simulink model "TPS_SWC"  (R2022b)
settings: Solver=FixedStepDiscrete  StartTime=0.0  StopTime=10.0  FixedStep=0.1  RelTol=1e-3
libraries: pil_lib x1
settings Model: Creator=Abdelrhman Shaban  LastModifiedBy=Abdelrhman Shaban
settings OptimizationCC: DefaultParameterBehavior=Inlined  UseDivisionForNetSlopeComputation=on  GainParamInheritBuiltInType=on  UseFloatMulNetSlope=on  InlineInvariantSignals=on  PassReuseOutputArgsAs=Individual arguments  ZeroExternalMemoryAtStartup=off  ZeroInternalMemoryAtStartup=off  NoFixptDivByZeroProtection=on  EfficientFloat2IntCast=on  LifeSpan=1  OptimizeBlockOrder=speed  DifferentSizesBufferReuse=on  EfficientTunableParamExpr=on
settings DebuggingCC: ParameterTunabilityLossMsg=error
settings HardwareCC: ProdLongLongMode=on
settings SFSimCC: MATLABDynamicMemAlloc=off
settings RTWCC: Description=Embedded Coder  SystemTargetFile=ert.tlc  TemplateMakefile=ert_default_tmf  CreateSILPILBlock=SIL
settings CodeAppCC: ForceParamTrailComments=on  IgnoreCustomStorageClasses=off  OperatorAnnotations=on  SimulinkDataObjDesc=on  SFDataObjDesc=on  CustomSymbolStrGlobalVar=rt$N$M  CustomSymbolStrType=$N$M  CustomSymbolStrFcn=$N$M$F  CustomSymbolStrMacro=$N$M  InsertBlockDesc=on
settings ERTTargetCC: TargetLangStandard=C99 (ISO)  GenerateSampleERTMain=on  IncludeMdlTerminateFcn=off  CombineSignalStateStructs=on  SuppressErrorStatus=on  SupportAbsoluteTime=off  SupportComplex=off  InlinedParameterPlacement=NonHierarchical  ERTCustomFileTemplate=example_file_process.tlc  ERTFilePackagingFormat=CompactWithDataFile

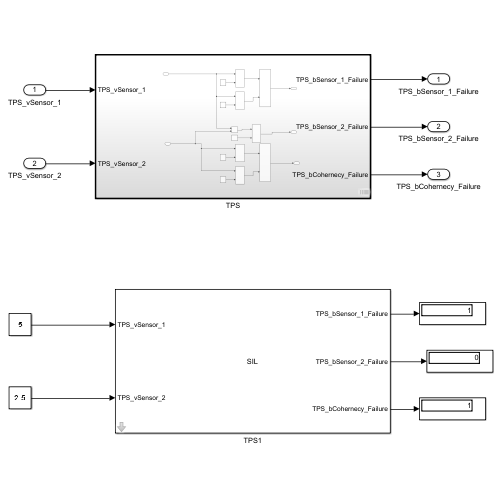
[thumbnail: Simulink's stored preview of the top-level diagram]
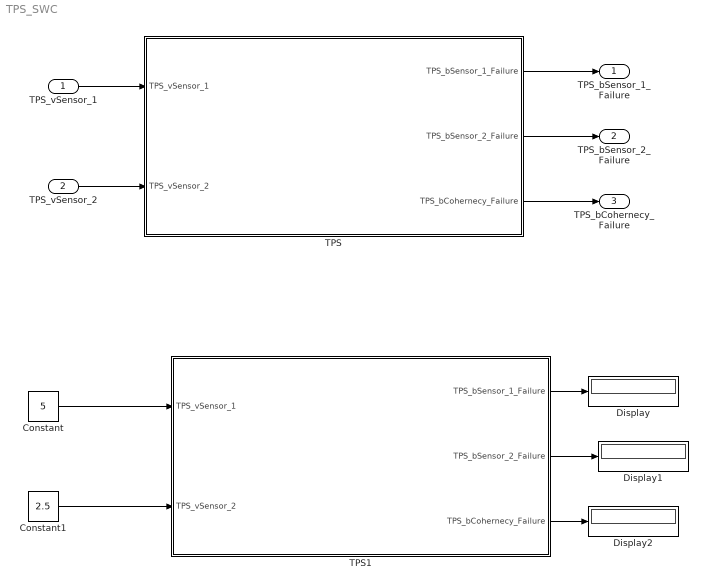
== system TPS_SWC ==
  TPS_vSensor_1 : Inport  OutDataTypeStr=single
  TPS_vSensor_2 : Inport  Port=2
  Constant : Constant  Value=5  OutDataTypeStr=single
  Constant1 : Constant  Value=2.5  OutDataTypeStr=single
  Display : Display
  Display1 : Display
  Display2 : Display
  TPS : Subsystem  TreatAsAtomicUnit=on
  TPS1 : Subsystem  Tag=__SL_testing_harness_stub_  DialogController=pil_create_dialog  LoadFcn=|
      | try
      |    if ~strcmp(rtw.pil.getPILVersion, '9.13 (R2022b)_15')
      |       set_param(gcb, 'DialogController', '');
      |       set_param(gcb, 'DialogControllerArgs', '');
      |    end
      | catch e
      |       set_param(gcb, 'DialogController', '');
      |       set_param(gcb, 'DialogControllerArgs', '');
      | end
      mask help: PIL:pil:XILBlockMaskDesc
      mask Display: disp('SIL');
  TPS_bSensor_1_Failure : Outport
  TPS_bSensor_2_Failure : Outport  Port=2
  TPS_bCohernecy_Failure : Outport  Port=3
  wires:
  TPS_vSensor_1/1 -> TPS/1(TPS_vSensor_1)
  TPS_vSensor_2/1 -> TPS/2(TPS_vSensor_2)
  TPS/1(TPS_bSensor_1_Failure) -> TPS_bSensor_1_Failure/1
  TPS/2(TPS_bSensor_2_Failure) -> TPS_bSensor_2_Failure/1
  TPS/3(TPS_bCohernecy_Failure) -> TPS_bCohernecy_Failure/1
  Constant/1 -> TPS1/1(TPS_vSensor_1)
  Constant1/1 -> TPS1/2(TPS_vSensor_2)
  TPS1/1(TPS_bSensor_1_Failure) -> Display/1
  TPS1/2(TPS_bSensor_2_Failure) -> Display1/1
  TPS1/3(TPS_bCohernecy_Failure) -> Display2/1

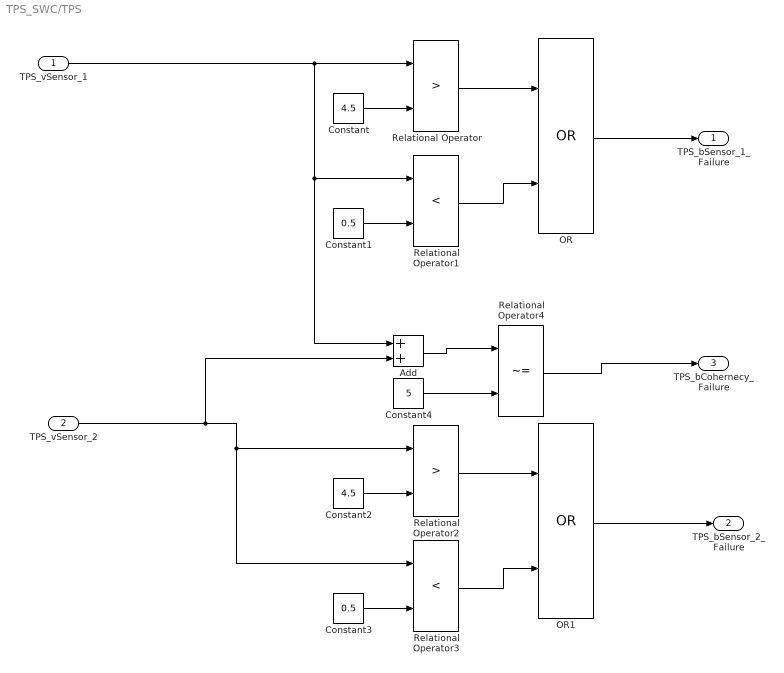
== system TPS_SWC/TPS ==
  TPS_vSensor_1 : Inport  OutDataTypeStr=single
  TPS_vSensor_2 : Inport  Port=2  OutDataTypeStr=single
  Add : Sum
  Constant : Constant  Value=4.5
  Constant1 : Constant  Value=0.5
  Constant2 : Constant  Value=4.5
  Constant3 : Constant  Value=0.5
  Constant4 : Constant  Value=5
  OR : Logic  Operator=OR  AllPortsSameDT=off  OutDataTypeStr=boolean
  OR1 : Logic  Operator=OR  AllPortsSameDT=off  OutDataTypeStr=boolean
  Relational Operator : RelationalOperator  Operator=>  OutDataTypeStr=boolean  RndMeth=Simplest  InputSameDT=off
  Relational Operator1 : RelationalOperator  Operator=<  OutDataTypeStr=boolean  RndMeth=Simplest  InputSameDT=off
  Relational Operator2 : RelationalOperator  Operator=>  OutDataTypeStr=boolean  RndMeth=Simplest  InputSameDT=off
  Relational Operator3 : RelationalOperator  Operator=<  OutDataTypeStr=boolean  RndMeth=Simplest  InputSameDT=off
  Relational Operator4 : RelationalOperator  Operator=~=  OutDataTypeStr=boolean  RndMeth=Simplest  InputSameDT=off
  TPS_bSensor_1_Failure : Outport  OutDataTypeStr=boolean
  TPS_bSensor_2_Failure : Outport  Port=2  OutDataTypeStr=boolean
  TPS_bCohernecy_Failure : Outport  Port=3  OutDataTypeStr=boolean
  wires:
  TPS_vSensor_1/1 -> Add/1, Relational Operator1/1, Relational Operator/1
  Constant/1 -> Relational Operator/2
  Constant1/1 -> Relational Operator1/2
  Relational Operator/1 -> OR/1
  Relational Operator1/1 -> OR/2
  OR/1 -> TPS_bSensor_1_Failure/1
  OR1/1 -> TPS_bSensor_2_Failure/1
  Relational Operator3/1 -> OR1/2
  Relational Operator2/1 -> OR1/1
  Constant3/1 -> Relational Operator3/2
  Constant2/1 -> Relational Operator2/2
  TPS_vSensor_2/1 -> Add/2, Relational Operator2/1, Relational Operator3/1
  Add/1 -> Relational Operator4/1
  Constant4/1 -> Relational Operator4/2
  Relational Operator4/1 -> TPS_bCohernecy_Failure/1

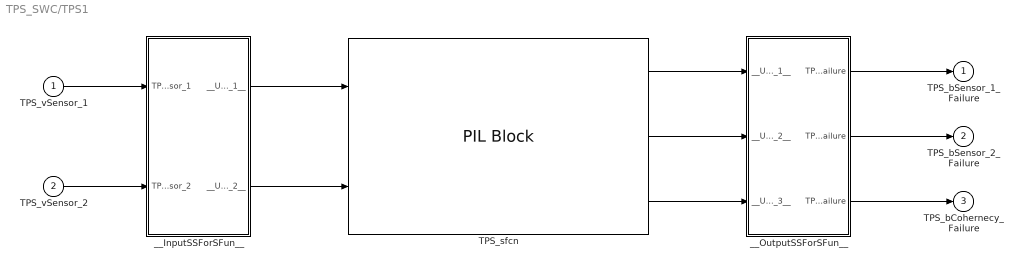
== system TPS_SWC/TPS1 ==
  TPS_vSensor_1 : Inport  OutDataTypeStr=single
  TPS_vSensor_2 : Inport  Port=2  OutDataTypeStr=single
  TPS_sfcn : pil_lib/PIL Block  SimulationMode=SIL  IsTopModelPIL=off  CodeDir=TPS_ert_rtw  AnchorDir=H:\AbdelrhmanWorkSpace\OSAcademy\Diploma\MBD_Diploma\6_System_Modeling\System_Modeling_Session_2\TechnicalPart\1_APP_Coherency  ConfigName=Software-in-the-Loop (SIL)  XrelIsTopModelCode=on  XrelIsReusable=off  XrelDWorkNames={}  XrelDWorkTypes={}  XrelModelArgVals={}  XrelOrderedParamNames={}
  __InputSSForSFun__ : Subsystem
  __OutputSSForSFun__ : Subsystem
  TPS_bSensor_1_Failure : Outport  OutDataTypeStr=boolean
  TPS_bSensor_2_Failure : Outport  Port=2  OutDataTypeStr=boolean
  TPS_bCohernecy_Failure : Outport  Port=3  OutDataTypeStr=boolean
  wires:
  __OutputSSForSFun__/3(TPS_bCohernecy_Failure) -> TPS_bCohernecy_Failure/1
  __OutputSSForSFun__/2(TPS_bSensor_2_Failure) -> TPS_bSensor_2_Failure/1
  __OutputSSForSFun__/1(TPS_bSensor_1_Failure) -> TPS_bSensor_1_Failure/1
  TPS_sfcn/3 -> __OutputSSForSFun__/3(__UniqueInportName__3__)
  TPS_sfcn/2 -> __OutputSSForSFun__/2(__UniqueInportName__2__)
  TPS_sfcn/1 -> __OutputSSForSFun__/1(__UniqueInportName__1__)
  __InputSSForSFun__/2(__UniqueOutportName__2__) -> TPS_sfcn/2
  __InputSSForSFun__/1(__UniqueOutportName__1__) -> TPS_sfcn/1
  TPS_vSensor_2/1 -> __InputSSForSFun__/2(TPS_vSensor_2)
  TPS_vSensor_1/1 -> __InputSSForSFun__/1(TPS_vSensor_1)

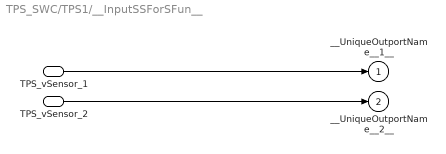
== system TPS_SWC/TPS1/__InputSSForSFun__ ==
  TPS_vSensor_1 : Inport  OutDataTypeStr=single
  TPS_vSensor_2 : Inport  Port=2  OutDataTypeStr=single
  __UniqueOutportName__1__ : Outport
  __UniqueOutportName__2__ : Outport  Port=2
  wires:
  TPS_vSensor_2/1 -> __UniqueOutportName__2__/1
  TPS_vSensor_1/1 -> __UniqueOutportName__1__/1

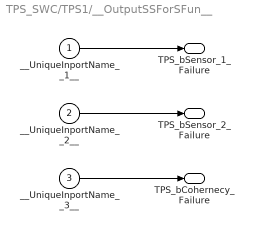
== system TPS_SWC/TPS1/__OutputSSForSFun__ ==
  __UniqueInportName__1__ : Inport
  __UniqueInportName__2__ : Inport  Port=2
  __UniqueInportName__3__ : Inport  Port=3
  TPS_bSensor_1_Failure : Outport  OutDataTypeStr=boolean
  TPS_bSensor_2_Failure : Outport  Port=2  OutDataTypeStr=boolean
  TPS_bCohernecy_Failure : Outport  Port=3  OutDataTypeStr=boolean
  wires:
  __UniqueInportName__3__/1 -> TPS_bCohernecy_Failure/1
  __UniqueInportName__2__/1 -> TPS_bSensor_2_Failure/1
  __UniqueInportName__1__/1 -> TPS_bSensor_1_Failure/1
